simulink model "DCDCconverter"  (R2012b)
settings: Solver=ode3  StartTime=0.0  StopTime=inf  FixedStep=Tsample_simulink  RelTol=1e-3
PostLoadFcn:
  | , if any(exist('dsrtsu_mdlpostloadfcn', 'file') == [2, 3, 6]), try dsrtsu_mdlpostloadfcn('Execute', bdroot); catch fprintf('Error in PostLoadFcn (dsrtsu_mdlpostloadfcn) for model "%s":\n %s\n', bdroot, lasterr); end, end,
InitFcn:
  | load('../sim/me547_based_PI_controller_v3_saved_state.mat');
  | load('../sim/RuleBasedControlData_LeadAcid_48V_25C.mat');
undefined symbols (not defined in the file): BatVoltageLowerThresh, BatVoltageUpperThresh, C, DiscIntNeverNeededParam, Ea, fdesignblkfcn, gcbh, Icommand_Limit, Ireg_Integ_Limit, Kp_vc, MaxBatCurrent, MaxBatVoltage, MaxTemperature, MaxUCCurrent, MaxUCVoltage, Ra, RuleBasedControlHESSPowerValues, RuleBasedControlLUTValues, RuleBasedControlUCVoltageValues, TDelay_UltracapacitorRelay, Ts, Ts2, Tsample_simulink, UCVoltageLowerThresh, UCVoltageUpperThresh, Vbat, Vrail_rated
libraries: xpclib x35, rtilib1103 x8, dspsigops x5
(part 9 of 10)

== stateflow chart DCDCconverter/Supervisory Control State Machine ==
  state InitState
    entry:
    delta_Voltage = 0.1
    VoltageCommand = Average_UCVoltage
    EnableVoltageCommand = 0
  state ChargeDownState
    during:
    VoltageCommand = UCVoltageUpperThresh - delta_Voltage
    EnableVoltageCommand = 1
  state CurrentControlState
    during:
    EnableVoltageCommand = 0
  state ChargeUpState
    during:
    VoltageCommand = UCVoltageLowerThresh + delta_Voltage
    EnableVoltageCommand = 1
  (default) -> InitState
  InitState -> ChargeDownState [order 2] : [( Average_UCVoltage >= UCVoltageUpperThresh ...
      | || Average_BatVoltage <= BatVoltageLowerThresh)...
      | && AutomaticControllerEnable == 1]
  InitState -> ChargeUpState [order 1] : [( Average_UCVoltage <= UCVoltageLowerThresh ...
      | || Average_BatVoltage >= BatVoltageUpperThresh)...
      | && AutomaticControllerEnable == 1]
  ChargeUpState -> InitState [order 2] : [AutomaticControllerEnable==0]
  ChargeDownState -> InitState [order 2] : [AutomaticControllerEnable==0]
  CurrentControlState -> InitState [order 3] : [AutomaticControllerEnable==0]
  InitState -> CurrentControlState [order 3] : [(Average_UCVoltage < UCVoltageUpperThresh ...
      | && Average_UCVoltage > UCVoltageLowerThresh ...
      | && Average_BatVoltage > BatVoltageLowerThresh ...
      | && Average_BatVoltage < BatVoltageUpperThresh)...
      | && AutomaticControllerEnable==1]
  CurrentControlState -> ChargeDownState [order 1] : [ (Average_UCVoltage >= UCVoltageUpperThresh ...
      | || UCVoltage_next_predicted >= UCVoltageUpperThresh ...
      | || Average_BatVoltage <= BatVoltageLowerThresh) ...
      | && UCCurrentCommand >= 0]
  ChargeDownState -> CurrentControlState [order 1] : [UCCurrentCommand < 0]
  CurrentControlState -> ChargeUpState [order 2] : [ (Average_UCVoltage <= UCVoltageLowerThresh ...
      | || UCVoltage_next_predicted <= UCVoltageLowerThresh ...
      | || Average_BatVoltage >= BatVoltageUpperThresh) ...
      | && UCCurrentCommand <= 0]
  ChargeUpState -> CurrentControlState [order 1] : [UCCurrentCommand > 0]
  data: Average_UCVoltage input; Average_BatVoltage input; UCCurrentCommand input; UCVoltage_next_predicted input; VoltageCommand output double; EnableVoltageCommand output double; BatVoltageLowerThresh input double; BatVoltageUpperThresh input double; UCVoltageLowerThresh input double; UCVoltageUpperThresh input double; delta_Voltage local double; AutomaticControllerEnable input; Kp_vc input

== stateflow chart DCDCconverter/System Configuration State Machine1 ==
  state Off
    entry:
    IGBT_Top_State = 0
    IGBT_Bot_State = 0
    AutomaticController = 0
    ChargingRelay = 0
    DischargingRelay = 1
    BatteryRelay = 0
    UltracapacitorRelay = 0
    dVrail_dT_threshold = 0.01
  state DischargingRail
    during:
    IGBT_Top_State = 0
    IGBT_Bot_State = 0
    AutomaticController = 0
    ChargingRelay = 0
    DischargingRelay = 1
    BatteryRelay = 0
    UltracapacitorRelay = 0
  state ChargingRail
    during:
    IGBT_Top_State = 0
    IGBT_Bot_State = 0
    AutomaticController = 0
    ChargingRelay = 1
    DischargingRelay = 0
    BatteryRelay = 0
    UltracapacitorRelay = 0
  state FinishedCharging
    during:
    IGBT_Top_State = 0
    IGBT_Bot_State = 0
    AutomaticController = 0
    ChargingRelay = 0
    DischargingRelay = 0
    BatteryRelay = 0
    UltracapacitorRelay = 0
  state AutomaticControlMode
    during:
    IGBT_Top_State = 1
    IGBT_Bot_State = 1
    AutomaticController = 1
    ChargingRelay = 0
    DischargingRelay = 0
    BatteryRelay = 1
    UltracapacitorRelay = 1
  state ManualBuckMode
    during:
    IGBT_Top_State = 2
    IGBT_Bot_State = 0
    AutomaticController = 0
    ChargingRelay = 0
    DischargingRelay = 0
    BatteryRelay = 1
    UltracapacitorRelay = 1
  state ManualBoostMode
    during:
    IGBT_Top_State = 0
    IGBT_Bot_State = 2
    AutomaticController = 0
    ChargingRelay = 0
    DischargingRelay = 0
    BatteryRelay = 1
    UltracapacitorRelay = 1
  (default) -> Off
  DischargingRail -> Off [order 2] : [Vrail <= Vrail_rated*0.15 && abs(dVrail_dT) <= dVrail_dT_threshold]
  Off -> ChargingRail : [TurnOnSystem == 1 && Error == 0]
  DischargingRail -> ChargingRail [order 1] : [TurnOnSystem == 1 && Error == 0]
  ChargingRail -> DischargingRail [order 2] : [Error == 1 || TurnOnSystem == 0]
  FinishedCharging -> DischargingRail [order 2] : [Error == 1 || TurnOnSystem == 0]
  ChargingRail -> FinishedCharging [order 1] : [Vrail >= Vrail_rated*0.85 && abs(dVrail_dT) <= dVrail_dT_threshold]
  ManualBuckMode -> DischargingRail [order 3] : [Error == 1 || TurnOnSystem == 0]
  ManualBoostMode -> DischargingRail [order 3] : [Error == 1 || TurnOnSystem == 0]
  AutomaticControlMode -> DischargingRail [order 3] : [Error == 1 || TurnOnSystem == 0]
  FinishedCharging -> ManualBuckMode [order 4] : [EnableAutomaticControl == 0 ...
      | && ManualControlBuckMode == 1]
  FinishedCharging -> ManualBoostMode [order 3] : [EnableAutomaticControl == 0 ...
      | && ManualControlBuckMode == 0]
  FinishedCharging -> AutomaticControlMode [order 1] : [EnableAutomaticControl == 1]
  ManualBoostMode -> AutomaticControlMode [order 2] : [EnableAutomaticControl == 1]
  ManualBuckMode -> ManualBoostMode [order 1] : [ManualControlBuckMode == 0]
  AutomaticControlMode -> ManualBoostMode [order 1] : [EnableAutomaticControl == 0 &&...
      | ManualControlBuckMode == 0]
  ManualBoostMode -> ManualBuckMode [order 1] : [ManualControlBuckMode == 1]
  AutomaticControlMode -> ManualBuckMode [order 2] : [EnableAutomaticControl == 0 && ManualControlBuckMode == 1]
  ManualBuckMode -> AutomaticControlMode [order 2] : [EnableAutomaticControl == 1]
  data: TurnOnSystem input; EnableAutomaticControl input; ManualControlBuckMode input; Error input; IGBT_Top_State output; IGBT_Bot_State output; Vrail input; dVrail_dT input; Vrail_rated input; AutomaticController output boolean; UltracapacitorRelay output double; ChargingRelay output double; DischargingRelay output double; BatteryRelay output double; dVrail_dT_threshold local double
